simulink model "crpm"  (R2020a)
settings: Solver=VariableStepAuto  StartTime=0.0  StopTime=10.0  RelTol=1e-3
libraries: simrfV2elements x1
settings Model: Creator=MAC  LastModifiedBy=MAC

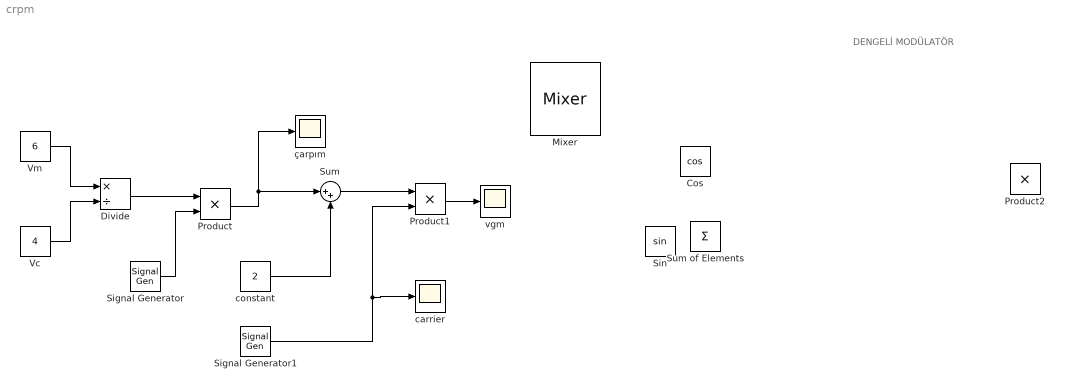
== system crpm ==
  note: DENGELİ MODÜLATÖR
  Cos : Trigonometry  Operator=cos
  Divide : Product  Inputs=*/
  Mixer : simrfV2elements/Mixer  classname=mixer  Source_linear_gain=Available power gain  linear_gain=0 dB  Zin=50  Zout=50  ZLO=inf  Source_Poly=Odd order  Poly_Coeffs=[0 1]  IPType=Output  IP2=Inf dBm  IP3=Inf dBm  P1dB=Inf dBm  Psat=Inf dBm  Gcomp=Inf dBm  NF=0  InternalGrounding=on
      settings: SourceProductBaseCode=RB
  Product : Product
  Product1 : Product
  Product2 : Product
  Signal Generator : SignalGenerator  Units=rad/sec
  Signal Generator1 : SignalGenerator  Units=rad/sec
  Sin : Trigonometry
  Sum : Sum  Inputs=|++
  Sum of Elements : Sum  Inputs=+
  Vc : Constant  Value=4
  Vm : Constant  Value=6
  carrier : Scope
  constant : Constant  Value=2
  vgm : Scope
  çarpım : Scope
  wires:
  Vm/1 -> Divide/1
  Vc/1 -> Divide/2
  Divide/1 -> Product/1
  Signal Generator/1 -> Product/2
  Product/1 -> çarpım/1, Sum/1
  constant/1 -> Sum/2
  Sum/1 -> Product1/1
  Signal Generator1/1 -> carrier/1, Product1/2
  Product1/1 -> vgm/1
